simulink model "mech_rolling_sphere"  (Simulink 6.0)
settings: Solver=ode45  StartTime=0.0  StopTime=40  RelTol=1e-3
undefined symbols (not defined in the file or in its folder): m, rad, s, sigbuilder_block
libraries: mblibv1 x11
settings Model: Creator=gwood  LastModifiedBy=batserve  ExtModeAutoUpdateStatusClock=off
settings DataIOCC: SignalLoggingName=sigsOut  OutputOption=SpecifiedOutputTimes  OutputTimes=[0:0.1:40]
settings DebuggingCC: CheckExecutionContextPreStartOutputMsg=on  CheckExecutionContextRuntimeOutputMsg=on  SolverPrmCheckMsg=none
settings HardwareCC: TargetUnknown=on
settings CodeAppCC: MangleLength=5
settings SimMechanicsCC: VisOnUpdateDiagram=on  VisDuringSimulation=on  VisConfigFile=mech_rolling_sphere.mat

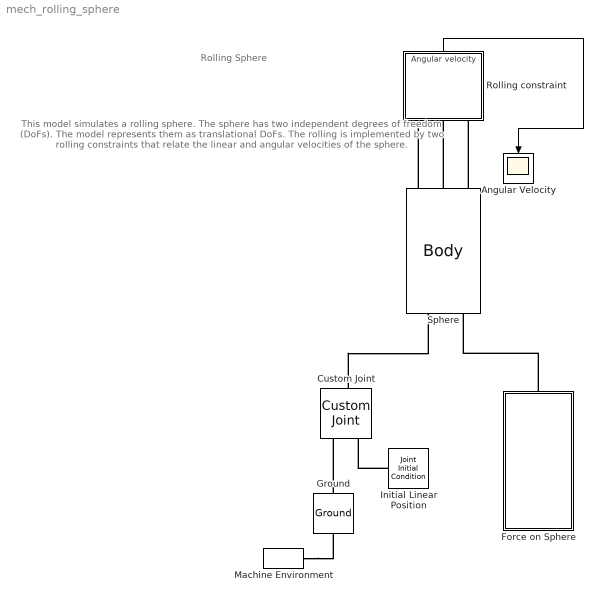
== system mech_rolling_sphere ==
  note: Rolling Sphere
  note: This model simulates a rolling sphere.  The sphere has
      | two independent degrees of freedom (DoFs).
      | The model represents them as translational DoFs.
      | The rolling is implemented by two rolling constraints
      | that relate the linear and angular velocities
      | of the sphere.
  Angular Velocity : Scope
      settings: Orientation=down  TimeRange=40  YMin=-0.5  YMax=1
  Custom Joint : mblibv1/Joints/Custom Joint  Orientation=up  PhysicalDomain=mechanical  SubClassName=custom_joint  LeftPortType=blob  RightPortType=blob  LConnTagsString=__newl0|SA1  RConnTagsString=__newr0  NumSAPorts=1  CutJoint=off  MarkAsCut=off  Primitives=prismatic_prismatic_spherical  PrimitiveProps=P1$WORLD$[1 0 0]$prismatic#P2$WORLD$[0 1 0]$prismatic#S$WORLD$[0 0 1]$spherical  DialogClass=JointBlock
  Force on Sphere : Subsystem  Orientation=up
  Ground : mblibv1/Bodies/Ground  Orientation=up  Opaque=on  LeftPortType=env  RightPortType=workingframe  PhysicalDomain=Mechanical  DialogClass=GroundBlock  CoordPosition=[0 0 1]  CoordPositionUnits=m  StateVectorMgrId=-1  MachineId=[0 0]  ShowEnvPort=on
  Initial Linear Position : mblibv1/Sensors &  Actuators/Joint Initial Condition  Orientation=left  Opaque=on  PhysicalDomain=Mechanical  DialogClass=InitialConditionBlock  InitialConditions=P1$true$0$m$rad$1$cm/s$rad/s#P2$true$0$m$rad$1$cm/s$rad/s#P3$false$0$m$rad$0$m/s$rad/s#R1$false$0$m$rad$0$m/s$rad/s#R2$false$0$m$rad$0$m/s$rad/s#R3$false$0$m$rad$0$m/s$rad/s#S$false$0$m$rad$0$m/s$rad/s
  Machine Environment : mblibv1/Bodies/Machine Environment  Tag=Factory ground  DialogController=MECH.DialogSource  Opaque=on  PortType=env  PhysicalDomain=Mechanical  DialogTemplateClass=MECH.MachineEnvironment  SyncWhenCopied=off  Gravity=[0 0 -9.81]  GravityUnits=m/s^2  GravityAsSignal=off  Dimensionality=3D Only  AnalysisType=Forward dynamics  LinearAssemblyTolerance=1e-3  LinearAssemblyToleranceUnits=m  AngularAssemblyTolerance=1e-3  AngularAssemblyToleranceUnits=rad  ConstraintSolverType=Stabilizing  ConstraintRelTolerance=1e-4  ConstraintAbsTolerance=1e-4  UseRobustSingularityHandling=off  StatePerturbationType=Fixed  PerturbationSize=1e-5  VisualizeMachine=on
  Rolling constraint : Subsystem  Orientation=up
  Sphere : mblibv1/Bodies/Body  Orientation=up  PhysicalDomain=mechanical  SubClassName=Unknown  LeftPortType=workingframe  RightPortType=workingframe  LConnTagsString=CS1|CS5  RConnTagsString=CS3|CS4|CS2  DialogClass=MechanicalBodyBlock  Mass=1  MassUnits=kg  InertiaUnits=kg*m^2  Inertia=(2/5)*eye(3)  Shape=Cylinder  ShapeDims=[1 1]  ShapeUnits=m  ShapeUse=false  Density=1  DensityUnits=kg/m^3  DensityUse=false  CG=Left$CG$[0 0 0]$CS1$CS1$m$[0 0 0]$Euler X-Y-Z$deg$WORLD$false  WorkingFrames=Left$CS1$[0 0 0]$ADJOINING$ADJOINING$m$[0 0 0]$Euler X-Y-Z$deg$WORLD$true#Right$CS3$[0 0 0]$CS1$CS1$m$[0 0 0]$Euler X-Y-Z$deg$WORLD$true#Right$CS4$[0 0 0]$CS1$CS1$m$[0 0 0]$Euler X-Y-Z$deg$WORLD$true#Right$CS2$[0 0 0]$CS1$CS1$m$[0 0 0]$Euler X-Y-Z$deg$WORLD$true#Left$CS5$[0 0 0]$CS1$CS1$m$[0 0 0]$Euler X-Y-Z$deg$WORLD$true
  wires:
  Rolling constraint/1(Angular velocity) -> Angular Velocity/1
  connections:
  Ground/RConn1 -- Custom Joint/LConn1
  Custom Joint/RConn1 -- Sphere/LConn1
  Initial Linear Position/RConn1 -- Custom Joint/LConn2
  Sphere/RConn3 -- Rolling constraint/LConn3
  Sphere/RConn2 -- Rolling constraint/LConn2
  Force on Sphere/RConn1 -- Sphere/LConn2
  Sphere/RConn1 -- Rolling constraint/LConn1
  Machine Environment/RConn1 -- Ground/LConn1

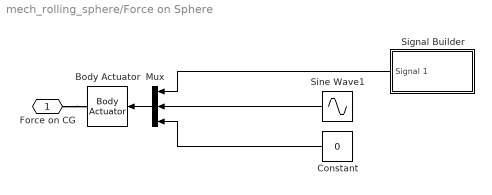
== system mech_rolling_sphere/Force on Sphere ==
  Body Actuator : mblibv1/Sensors &  Actuators/Body Actuator  Orientation=left  Opaque=on  PhysicalDomain=Mechanical  PortType=blob  ActuationStyle=Force  AngleUnits=deg  ArcVelocityUnits=deg/s  ArcAccelerationUnits=deg/s^2  CoordPositionUnits=m  VelocityUnits=m/s  AccelerationUnits=m/s^2  ForceUnits=N  TorqueUnits=N-m  ActiveIO=on  Width=3  DialogClass=MechanicalActuatorBlock  ReferenceFrame=Absolute (World)  Angle=off  CoordPosition=on  Force=on  Torque=off
  Constant : Constant  Orientation=left  Value=0
  Mux : Mux  Orientation=left  Inputs=3
  Signal Builder : Subsystem  Tag=STV Subsys  Orientation=left  LoadFcn=sigbuilder_block('load');  StartFcn=sigbuilder_block('start');  StopFcn=sigbuilder_block('stop');  ClipboardFcn=sigbuilder_block('clipboard');  mask(Sigbuilder block){}
      mask help: Sigbuilder GUI
      mask init:
      | if ~strcmp(get_param(bdroot(gcb),'SimulationStatus'),'stopped') tuvar = sigbuilder_block('maskInit'); end
      settings: CopyFcn=sigbuilder_block('copy');  DeleteFcn=sigbuilder_block('delete');  ModelCloseFcn=sigbuilder_block('modelClose');  PreSaveFcn=sigbuilder_block('preSave');  NameChangeFcn=sigbuilder_block('namechange');  OpenFcn=sigbuilder_block('open',[50 50 520 400 ]);  CloseFcn=sigbuilder_block('close');
      mask Display: plot(0,0,100,100,[10,10,40,40,10],[80,20,20,80,80],[40,10],[50,50], [40,27,10],[65,72,56],[40,25,25,10],[28,28,43,43]);
  Sine Wave1 : Sin  Orientation=left  Amplitude=0.1  Frequency=0.7  SampleTime=0
  Force on CG : PMIOPort  Port=1  Side=Right
  wires:
  Mux/1 -> Body Actuator/1
  Signal Builder/1(Signal 1) -> Mux/1
  Sine Wave1/1 -> Mux/2
  Constant/1 -> Mux/3
  connections:
  Force on CG/RConn1 -- Body Actuator/RConn1

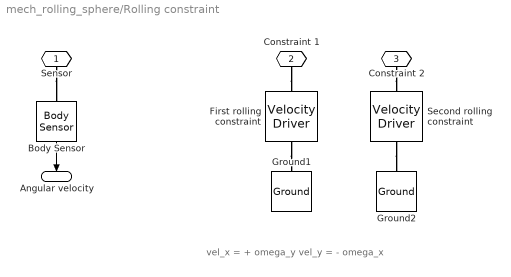
== system mech_rolling_sphere/Rolling constraint ==
  note: vel_x = + omega_y
      | vel_y = - omega_x
  Body Sensor : mblibv1/Sensors &  Actuators/Body Sensor  Orientation=down  Opaque=on  PhysicalDomain=Mechanical  PortType=blob  Muxed=on  Pose=off  Angle=on  AngleUnits=deg  ArcVelocity=on  ArcVelocityUnits=rad/s  ArcAcceleration=off  ArcAccelerationUnits=deg/s^2  CoordPosition=off  CoordPositionUnits=m  Velocity=off  VelocityUnits=m/s  Acceleration=off  AccelerationUnits=m/s^2  Quaternion=on  QuaternionDT=off  QuaternionDDT=off  QuaternionUnits=off  OutputVector=[ 3 ]  ActiveIO=on  Width=3  DialogClass=MechanicalSensorBlock  ReferenceFrame=Absolute (World)
  First rolling constraint : mblibv1/Constraints &  Drivers/Velocity Driver  Orientation=down  PhysicalDomain=mechanical  SubClassName=Unknown  LeftPortType=blob  RightPortType=blob  LConnTagsString=__newl0  RConnTagsString=__newr0  DialogClass=ConstantVelocityConstraint  NumSAPorts=0  Unit_V=m/s  Unit_Omega=rad/s  Coef_V_Base=[1 0 0]  Csys_V_Base=WORLD  Coef_Omega_Base=[0 -1 0]  Csys_Omega_Base=WORLD  Coef_V_Follower=[0 0 0]  Csys_V_Follower=WORLD  Coef_Omega_Follower=[0 0 0]  Csys_Omega_Follower=WORLD
  Ground1 : mblibv1/Bodies/Ground  Orientation=up  Opaque=on  LeftPortType=env  RightPortType=workingframe  PhysicalDomain=Mechanical  DialogClass=GroundBlock  CoordPosition=[0 0 0]  CoordPositionUnits=m  StateVectorMgrId=-1  MachineId=[0 0]  ShowEnvPort=off
  Ground2 : mblibv1/Bodies/Ground  Orientation=up  Opaque=on  LeftPortType=env  RightPortType=workingframe  PhysicalDomain=Mechanical  DialogClass=GroundBlock  CoordPosition=[0 0 0]  CoordPositionUnits=m  StateVectorMgrId=-1  MachineId=[0 0]  ShowEnvPort=off
  Second rolling constraint : mblibv1/Constraints &  Drivers/Velocity Driver  Orientation=down  PhysicalDomain=mechanical  SubClassName=Unknown  LeftPortType=blob  RightPortType=blob  LConnTagsString=__newl0  RConnTagsString=__newr0  DialogClass=ConstantVelocityConstraint  NumSAPorts=0  Unit_V=m/s  Unit_Omega=rad/s  Coef_V_Base=[0 1 0]  Csys_V_Base=WORLD  Coef_Omega_Base=[1 0 0]  Csys_Omega_Base=WORLD  Coef_V_Follower=[0 0 0]  Csys_V_Follower=WORLD  Coef_Omega_Follower=[0 0 0]  Csys_Omega_Follower=WORLD
  Sensor : PMIOPort  Orientation=down  Port=1  Side=Left
  Constraint 1 : PMIOPort  Orientation=down  Port=2  Side=Left
  Constraint 2 : PMIOPort  Orientation=down  Port=3  Side=Left
  Angular velocity : Outport  Orientation=down
  wires:
  Body Sensor/1 -> Angular velocity/1
  connections:
  First rolling constraint/RConn1 -- Ground1/RConn1
  Second rolling constraint/RConn1 -- Ground2/RConn1
  Constraint 2/RConn1 -- Second rolling constraint/LConn1
  Constraint 1/RConn1 -- First rolling constraint/LConn1
  Sensor/RConn1 -- Body Sensor/LConn1

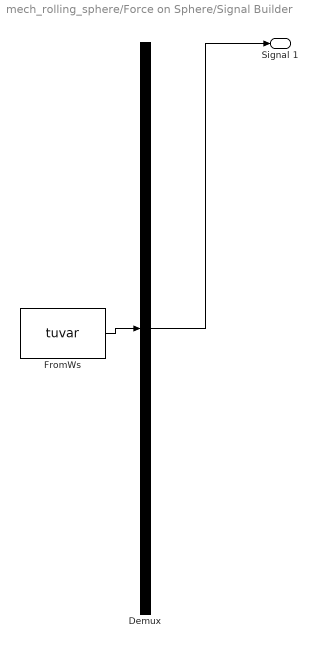
== system mech_rolling_sphere/Force on Sphere/Signal Builder ==
  Demux : Demux  Tag=STV Demux  Outputs=1
  FromWs : FromWorkspace  Tag=STV FromWs  VariableName=tuvar  SampleTime=0  SigBuilderData=DataTag0  VnvData=DataTag1
      SigBuilderData=|
      | channels.label = 'Signal 1'
      | channels.allXData = {[0 0.44 0.44 2.84 2.84 5.92 5.92 10]}
      | channels.allYData = {[0 0 0.5 0.5 -0.51 -0.51 0 0]}
      | dataSet.timeRange = [0 10]
      | dataSet.name = 'Group 1'
  Signal 1 : Outport  Tag=STV Outport
  wires:
  Demux/1 -> Signal 1/1
  FromWs/1 -> Demux/1
